simulink model "Reduce_Block_Diagram_1"  (R2024a)
settings: Solver=VariableStepAuto  StartTime=0.0  StopTime=10  RelTol=1e-3
values from neighbouring files (symbols this model uses):
  G1_den = [1 0 0]    [Reduce_Block_Diagram_1.m]
  G1_num = [1]    [Reduce_Block_Diagram_1.m]    (also in Reduce_Block_Diagram_2.m)
  G2_den = [1 1]    [Reduce_Block_Diagram_1.m]    (also in Reduce_Block_Diagram_2.m)
  G2_num = [1]    [Reduce_Block_Diagram_1.m]    (also in Reduce_Block_Diagram_2.m)
  G3_den = [1 0]    [Reduce_Block_Diagram_1.m]    (also in Reduce_Block_Diagram_2.m)
  G3_num = [1]    [Reduce_Block_Diagram_1.m]    (also in Reduce_Block_Diagram_2.m)
  H1_den = [1 0]    [Reduce_Block_Diagram_1.m]
  H1_num = [1]    [Reduce_Block_Diagram_1.m]
  H2_den = [1 -1]    [Reduce_Block_Diagram_1.m]
  H2_num = [1]    [Reduce_Block_Diagram_1.m]
  H3_den = [1 -2]    [Reduce_Block_Diagram_1.m]
  H3_num = [1]    [Reduce_Block_Diagram_1.m]

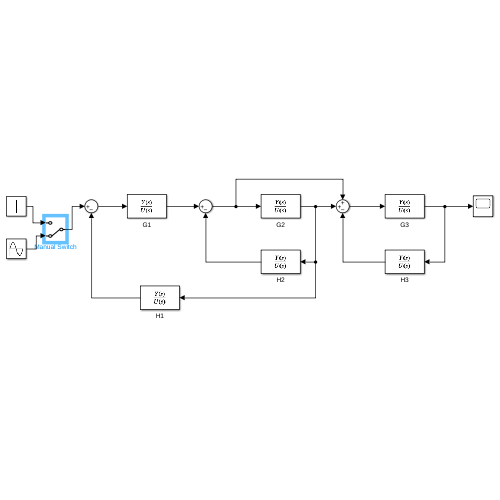
[thumbnail: Simulink's stored preview of the top-level diagram]
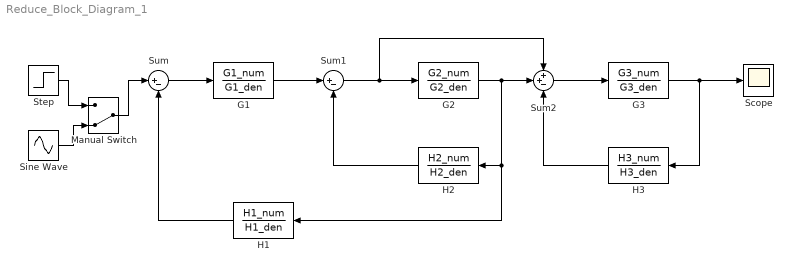
== system Reduce_Block_Diagram_1 ==
  G1 : TransferFcn  Numerator=G1_num  Denominator=G1_den
  G2 : TransferFcn  Numerator=G2_num  Denominator=G2_den
  G3 : TransferFcn  Numerator=G3_num  Denominator=G3_den
  H1 : TransferFcn  Numerator=H1_num  Denominator=H1_den
  H2 : TransferFcn  Numerator=H2_num  Denominator=H2_den
  H3 : TransferFcn  Numerator=H3_num  Denominator=H3_den
  Manual Switch : ManualSwitch  CurrentSetting=0
  Scope : Scope
  Sine Wave : Sin  SampleTime=0
  Step : Step  Time=0  SampleTime=0
  Sum : Sum  Inputs=|+-
  Sum1 : Sum  Inputs=|+-
  Sum2 : Sum  Inputs=++-
  wires:
  Step/1 -> Manual Switch/1
  Sum/1 -> G1/1
  H1/1 -> Sum/2
  G1/1 -> Sum1/1
  Sum1/1 -> Sum2/1, G2/1
  H2/1 -> Sum1/2
  G2/1 -> H1/1, H2/1, Sum2/2
  Sum2/1 -> G3/1
  H3/1 -> Sum2/3
  G3/1 -> H3/1, Scope/1
  Sine Wave/1 -> Manual Switch/2
  Manual Switch/1 -> Sum/1
